simulink model "CarHalf"  (R2018b)
settings: Solver=VariableStepAuto  StartTime=0.0  StopTime=10  MaxStep=0.001  RelTol=1e-3
values from neighbouring files (symbols this model uses):
  a = b    (= 1.5)    [CarQuarterParam.m]
  b = 1.5    [CarQuarterParam.m]
  Lamda = 1    [CarQuarterParam.m]
  speed = 2    [CarQuarterParam.m]
settings Model: Creator=Reece Bell  LastModifiedBy=Reece Bell

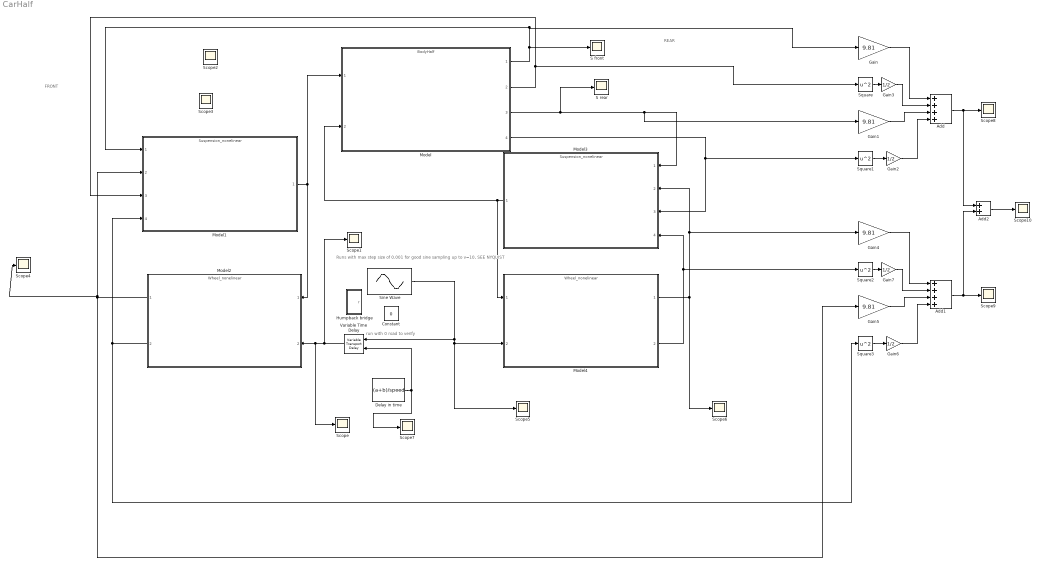
== system CarHalf ==
  note: Runs with max step size of 0.001 for good sine sampling up to v=10, SEE NYQUIST
  note: run with 0 road to verify
  note: REAR
  note: FRONT
  Add : Sum  Inputs=++++
  Add1 : Sum  Inputs=++++
  Add2 : Sum
  Constant : Constant  Value=0
  Delay in time : Constant  Value=(a+b)/speed
  Gain{,1,4..5} (4 alike) : Gain  Gain=9.81
  Gain{2..3,6..7} (4 alike) : Gain  Gain=1/2
  Humpback bridge : Subsystem  mask{h=2, L=20, v=speed}
      mask prompts: h "humpback height (m)"; L "humpback length (m)"; v "vehicle speed (m/s)"
  Model : ModelReference  ModelNameDialog=BodyHalf.slx  SimulationMode=Normal  ModelReferenceVersion=1.5
  Model1 : ModelReference  ModelNameDialog=Suspension_nonelinear.slx  SimulationMode=Normal  ModelReferenceVersion=1.10
  Model2 : ModelReference  ModelNameDialog=Wheel_nonelinear.slx  SimulationMode=Normal  ModelReferenceVersion=1.17
  Model3 : ModelReference  ModelNameDialog=Suspension_nonelinear.slx  SimulationMode=Normal  ModelReferenceVersion=1.10
  Model4 : ModelReference  ModelNameDialog=Wheel_nonelinear.slx  SimulationMode=Normal  ModelReferenceVersion=1.17
  S front : Scope
  S rear : Scope
  Scope{,1..10} (11 alike) : Scope
  Sine Wave : Sin  Frequency=(speed*2*pi)/Lamda  SampleTime=0
  Square{,1..3} (4 alike) : Math  Operator=square  SaturateOnIntegerOverflow=on
  Variable Time Delay : VariableTransportDelay  MaximumDelay=10
  wires:
  Model2/1 -> Gain5/1, Scope4/1, Model1/2
  Model2/2 -> Square3/1, Model1/4
  Model1/1 -> Model/1, Model2/1
  Model4/1 -> Gain4/1, Model3/2, Scope6/1
  Model4/2 -> Square2/1, Model3/4
  Variable Time Delay/1 -> Scope1/1, Scope/1, Model2/2
  Delay in time/1 -> Variable Time Delay/2, Scope7/1
  Model3/1 -> Model/2, Model4/1
  Sine Wave/1 -> Variable Time Delay/1, Scope5/1, Model4/2
  Gain1/1 -> Add/3
  Gain/1 -> Add/1
  Model/3 -> S rear/1, Gain1/1, Model3/1
  Gain2/1 -> Add/4
  Model/4 -> Square1/1, Model3/3
  Model/2 -> Square/1, Model1/3
  Square1/1 -> Gain2/1
  Square/1 -> Gain3/1
  Add/1 -> Add2/1, Scope8/1
  Gain3/1 -> Add/2
  Model/1 -> S front/1, Gain/1, Model1/1
  Gain7/1 -> Add1/2
  Add1/1 -> Add2/2, Scope9/1
  Gain6/1 -> Add1/4
  Gain4/1 -> Add1/1
  Gain5/1 -> Add1/3
  Square3/1 -> Gain6/1
  Square2/1 -> Gain7/1
  Add2/1 -> Scope10/1

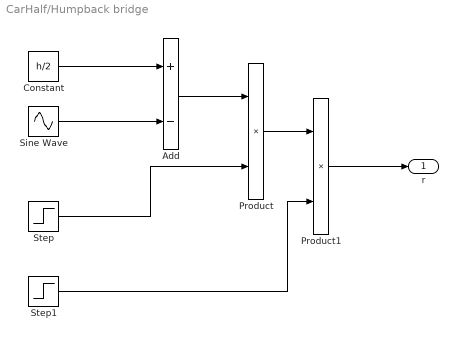
== system CarHalf/Humpback bridge ==
  Add : Sum  Inputs=+-
  Constant : Constant  Value=h/2
  Product : Product
  Product1 : Product
  Sine Wave : Sin  Amplitude=h/2  Frequency=2*pi*v/L  Phase=pi/2  SampleTime=0
  Step : Step  Time=2*L/v  SampleTime=0
  Step1 : Step  Time=3*L/v  Before=1  After=0  SampleTime=0
  r : Outport
  wires:
  Constant/1 -> Add/1
  Sine Wave/1 -> Add/2
  Add/1 -> Product/1
  Step/1 -> Product/2
  Product/1 -> Product1/1
  Step1/1 -> Product1/2
  Product1/1 -> r/1
